simulink model "Rayleigh_Fading_Channel"  (R2019a)
settings: Solver=VariableStepAuto  StartTime=0.0  StopTime=15.0  RelTol=1e-3
undefined symbols (not defined in the file or in its folder): doppler, magnitude
libraries: commdigbbndpm3 x2, dspsnks4 x1, dspvision x1, commutil2 x1, commchan3 x1
settings Model: Creator=surag  LastModifiedBy=surag

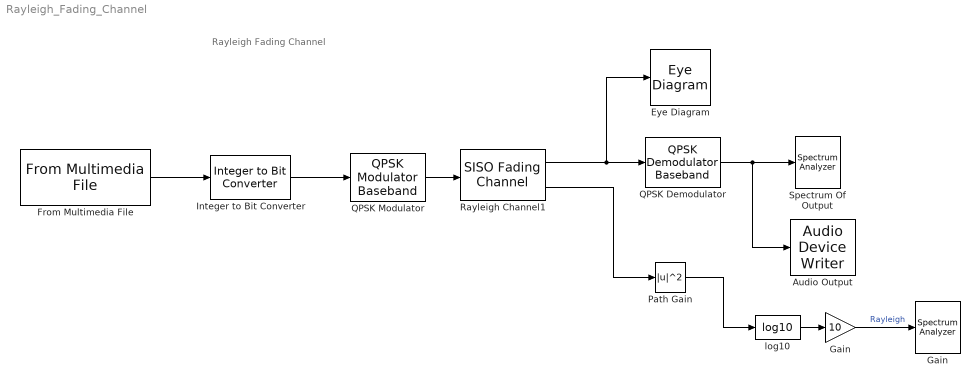
== system Rayleigh_Fading_Channel ==
  note: Rayleigh Fading Channel
  " Path Gain" : Math  Operator=magnitude^2  SaturateOnIntegerOverflow=on
  Audio Output : dspsnks4/Audio Device Writer  Driver=CoreAudio  Device=Default  InheritSampleRate=on  SampleRate=44100  BitDepth=16-bit integer  BufferSize=4096  NumBuffers=10  DefaultOutputChannelMapping=on  OutputChannelMapping=1:2  OutputNumUnderrunSamples=off  DriverIdx=5  DeviceWarnFlag=''
  Eye Diagram : EyeDiagram
  From Multimedia File : dspvision/From Multimedia File  inputFilename=/Users/surag/Downloads/audiotestfiles/sourceCode\sourceCode/WAV/IEEE Float/IEEE float mono 96kHz.wav  readRange=[1 Inf]  loop=on  numPlays=inf  outputStreams=Audio only  videoDataType=single  audioDataType=uint8  inheritSampleTime=on  userDefinedSampleTime=1/30  noAudioOutput=off  isIntensityVideo=off  fourcc=RGB  colorVideoFormat=Separate color signals  outputEOF=off  dataOrg=Column-major  audioFrameSize=1024  computeAudioFrameSize=off  outSamplingMode=Sample based
      settings: SourceProductName=DSP System Toolbox  SourceProductBaseCode=DS
  Gain : Gain  Gain=10  SaturateOnIntegerOverflow=on  OutDataTypeStr=Inherit: Same as input  ParamDataTypeStr=Inherit: Same as input
  "Gain " : SpectrumAnalyzer
  Integer to Bit Converter : commutil2/Integer to Bit Converter  nbits=8  signedInputValues=Unsigned  bitOrder=MSB first  outDtype=Inherit via internal rule
      settings: SourceProductName=Communications Toolbox
  "QPSK Demodulator " : commdigbbndpm3/QPSK Demodulator Baseband  OutType=Integer  DecType=Hard decision  VarSource=Dialog  Variance=1  Dec=Gray  Ph=pi/4  outDtype1=Inherit via internal rule  outDtype2=Inherit via internal rule  derotateFactorWordLen=16  derotateFactorDataTypeStr=Inherit: Same word length as input  derotateFactorLastDataTypeStr=Inherit: Same word length as input
      settings: SourceProductName=Communications Toolbox
  QPSK Modulator : commdigbbndpm3/QPSK Modulator Baseband  InType=Bit  Enc=Gray  Ph=pi/4  outDtype=double  outWordLen=16  outUDDataType=sfix(16)  outFracLenMode=Best precision  outFracLen=15  outDataTypeStr=double  outLastDataTypeStr=double
      settings: SourceProductName=Communications Toolbox
  Rayleigh Channel1 : commchan3/SISO Fading Channel  InheritSampleRate=on  SampleRate=1  PathDelays=[0 2e-07 4e-07 8e-07]  AveragePathGains=[0 -3 -6 -9]  NormalizePathGains=on  FadingDistribution=Rayleigh  KFactor=3  DirectPathDopplerShift=0  DirectPathInitialPhase=0  MaximumDopplerShift=10  DopplerSpectrum=doppler('Jakes')  ChannelInterpolationMethod=Polyphase  RandomStream=mt19937ar with seed  RandomNumGenerator=mt19937ar  Seed=12345  PathGainsOutputPort=on  ChannelFilterDelayOutputPort=off  SimulateUsing=Interpreted execution  Visualization=Doppler spectrum  PathsForDopplerDisplay=1  SamplesToDisplay=50%
      settings: SourceProductName=Communications Toolbox
  Spectrum Of Output : SpectrumAnalyzer
  log10 : Math  Operator=log10  SaturateOnIntegerOverflow=on
  wires:
  QPSK Modulator/1 -> Rayleigh Channel1/1
  Integer to Bit Converter/1 -> QPSK Modulator/1
  Rayleigh Channel1/1 -> Eye Diagram/1, "QPSK Demodulator "/1
  Gain/1 -> "Gain "/1  "Rayleigh"
  From Multimedia File/1 -> Integer to Bit Converter/1
  "QPSK Demodulator "/1 -> Spectrum Of Output/1, Audio Output/1
  Rayleigh Channel1/2 -> " Path Gain"/1
  log10/1 -> Gain/1
  " Path Gain"/1 -> log10/1
